simulink model "simple_lookuptable"  (R2024b)
settings: Solver=ode3  StartTime=0.0  StopTime=10.0  FixedStep=0.1  RelTol=1e-3
libraries: simulink x1
settings Model: Creator=balaj  LastModifiedBy=balaj

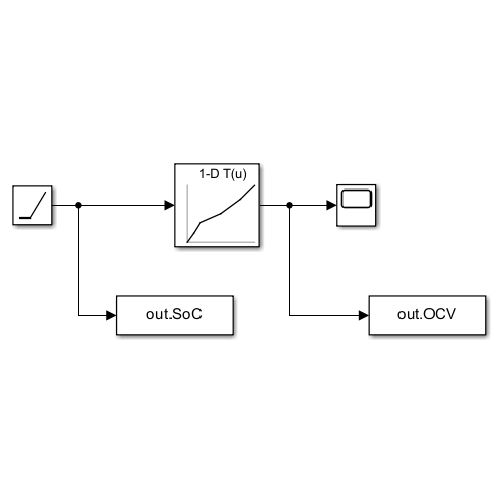
[thumbnail: Simulink's stored preview of the top-level diagram]
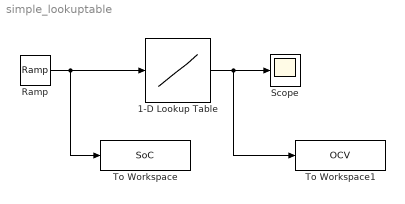
== system simple_lookuptable ==
  1-D Lookup Table : Lookup_n-D  NumberOfTableDimensions=1  BreakpointsForDimension1=[0 10 20 50 80 100]  Table=[3.0 3.2 3.4 3.6 3.9 4.2]  InternalRulePriority=Speed  RndMeth=Simplest
  Ramp : simulink/Sources/Ramp  slope=10  start=0  InitialOutput=0
  Scope : Scope
  To Workspace : ToWorkspace  VariableName=SoC  SaveFormat=Structure With Time  SampleTime=-1
  To Workspace1 : ToWorkspace  VariableName=OCV  SaveFormat=Structure With Time  SampleTime=-1
  wires:
  Ramp/1 -> To Workspace/1, 1-D Lookup Table/1
  1-D Lookup Table/1 -> To Workspace1/1, Scope/1
